simulink model "MagTest"  (R2021a)
settings: Solver=VariableStepAuto  StartTime=0.0  StopTime=10.0  RelTol=1e-3
libraries: simulink x3
settings Model: Creator=jmher  LastModifiedBy=jmher

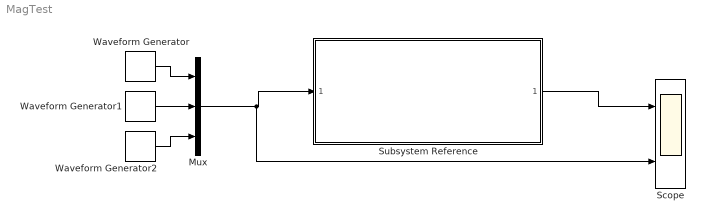
== system MagTest ==
  Mux : Mux  Inputs=3
  Scope : Scope  NumInputPorts=2
  Subsystem Reference : Subsystem  ReferencedSubsystem=Magnetometer
  Waveform Generator : simulink/Sources/Waveform Generator  OutMin=[]  OutMax=[]  OutDataTypeStr=double  SelectedSignal=1  Signals=sin(30e-6, 1, 0)  BlockNames=MultiportSwitch_73958a4ddd754e7  SampleTime=0.1
  Waveform Generator1 : simulink/Sources/Waveform Generator  OutMin=[]  OutMax=[]  OutDataTypeStr=double  SelectedSignal=1  Signals=sin(30e-6, 1, 0)  BlockNames=MultiportSwitch_c82bd7a658b84e3  SampleTime=0.1
  Waveform Generator2 : simulink/Sources/Waveform Generator  OutMin=[]  OutMax=[]  OutDataTypeStr=double  SelectedSignal=1  Signals=sin(30e-6, 1, 0)  BlockNames=MultiportSwitch_c0f71e69ba0d46c  SampleTime=0.1
  wires:
  Subsystem Reference/1 -> Scope/1
  Waveform Generator2/1 -> Mux/3
  Waveform Generator1/1 -> Mux/2
  Waveform Generator/1 -> Mux/1
  Mux/1 -> Scope/2, Subsystem Reference/1
